simulink model "EScooter_Context_Physical"  (R2025b)
settings: Solver=VariableStepAuto  StartTime=0.0  StopTime=10.0  RelTol=1e-3
settings Model: Creator=louis  LastModifiedBy=louis

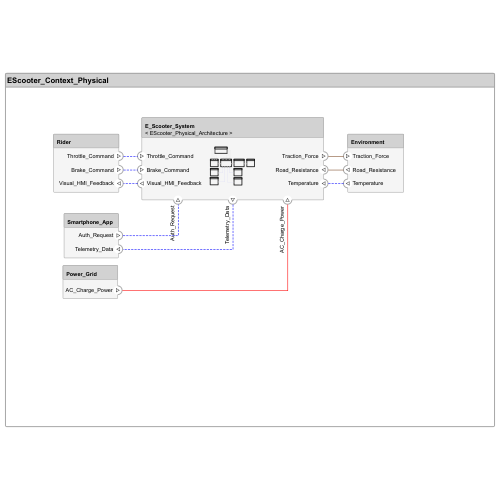
[thumbnail: Simulink's stored preview of the top-level diagram]
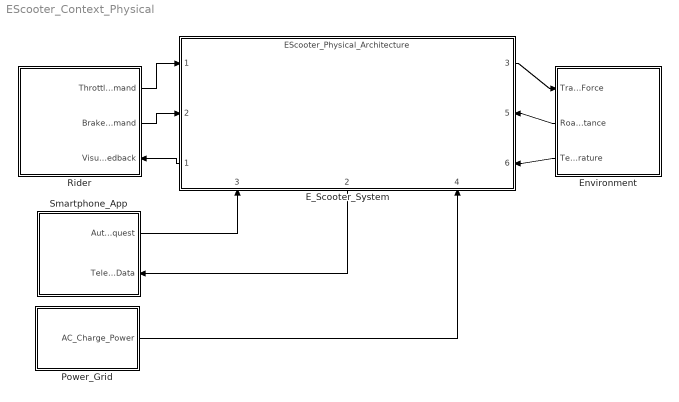
== system EScooter_Context_Physical ==
  E_Scooter_System : ModelReference  ModelNameDialog=EScooter_Physical_Architecture  SimulationMode=Normal  ModelReferenceVersion=1.35
      settings: PortSchema="{\"entries\":[{\"content\":{\"headerSize\":38,\"margin\":15,\"minimumSpacing\":25,\"sides\":[{\"content\":{\"connectorIds\":[\"In1\",\"In2\",\"Out1\"]},\"type\":\"ConnectorPlacement.EquallySpacedRectSide\",\"uuid\":\"e3bd6986-1133-4d24-a772-f86194006591\"},{\"content\":{\"connectorIds\":[\"Out3\",\"In5\",\"In6\"],\"side\":\"RIGHT\"},\"type\":\"ConnectorPlacement.EquallySpacedRectSide\",\"uuid\":\"35d8fe16-ac3e-4ad7-9024-4759d4f7a595\"},{\"content\":{\"side\":\"TOP\"},\"type\":\"ConnectorPlacement.EquallySpacedRectSide\",\"uuid\":\"5c4c1cf0-f549-46fb-a8e2-98c3709b9973\"},{\"content\":{\"connectorIds\":[\"In3\",\"Out2\",\"In4\"],\"side\":\"BOTTOM\"},\"type\":\"ConnectorPlacement.EquallySpacedRectSide\",\"uuid\":\"d5812157-23f3-4c6d-a0b8-9b10c8e876d4\"}]},\"type\":\"ConnectorPlacement.EquallySpacedConnector\",\"uuid\":\"87a80faf-9870-4a1b-94c7-6fcc75790299\"}],\"packageUris\":[\"http://schema.mathworks.com/mf0/Connector/R2020b\"],\"version\":\"1.0\"}"
  Environment : Subsystem
      settings: PortSchema="{\"entries\":[{\"content\":{\"headerSize\":26,\"margin\":15,\"minimumSpacing\":25,\"sides\":[{\"content\":{\"connectorIds\":[\"In1\",\"Out1\",\"Out2\"]},\"type\":\"ConnectorPlacement.EquallySpacedRectSide\",\"uuid\":\"144652b9-dd85-470f-8014-e792da2fa2ac\"},{\"content\":{\"side\":\"RIGHT\"},\"type\":\"ConnectorPlacement.EquallySpacedRectSide\",\"uuid\":\"d391e3f2-978f-4ccc-ab2b-52567d421a28\"},{\"content\":{\"side\":\"TOP\"},\"type\":\"ConnectorPlacement.EquallySpacedRectSide\",\"uuid\":\"a45f99b3-1281-4051-bb9b-2205db18ec2a\"},{\"content\":{\"side\":\"BOTTOM\"},\"type\":\"ConnectorPlacement.EquallySpacedRectSide\",\"uuid\":\"ad3f1504-e103-4633-a1e9-d1d529d4f8d7\"}]},\"type\":\"ConnectorPlacement.EquallySpacedConnector\",\"uuid\":\"69c8647b-5d40-4da9-a90b-a75e053ae147\"}],\"packageUris\":[\"http://schema.mathworks.com/mf0/Connector/R2020b\"],\"version\":\"1.0\"}"
  Power_Grid : Subsystem
      settings: PortSchema="{\"entries\":[{\"content\":{\"headerSize\":26,\"margin\":15,\"minimumSpacing\":25,\"sides\":[{\"content\":{},\"type\":\"ConnectorPlacement.EquallySpacedRectSide\",\"uuid\":\"144652b9-dd85-470f-8014-e792da2fa2ac\"},{\"content\":{\"connectorIds\":[\"Out1\"],\"side\":\"RIGHT\"},\"type\":\"ConnectorPlacement.EquallySpacedRectSide\",\"uuid\":\"d391e3f2-978f-4ccc-ab2b-52567d421a28\"},{\"content\":{\"side\":\"TOP\"},\"type\":\"ConnectorPlacement.EquallySpacedRectSide\",\"uuid\":\"a45f99b3-1281-4051-bb9b-2205db18ec2a\"}]},\"type\":\"ConnectorPlacement.EquallySpacedConnector\",\"uuid\":\"69c8647b-5d40-4da9-a90b-a75e053ae147\"}],\"packageUris\":[\"http://schema.mathworks.com/mf0/Connector/R2020b\"],\"version\":\"1.0\"}"
  Rider : Subsystem
      settings: PortSchema="{\"entries\":[{\"content\":{\"headerSize\":26,\"margin\":15,\"minimumSpacing\":25,\"sides\":[{\"content\":{},\"type\":\"ConnectorPlacement.EquallySpacedRectSide\",\"uuid\":\"144652b9-dd85-470f-8014-e792da2fa2ac\"},{\"content\":{\"connectorIds\":[\"Out2\",\"Out1\",\"In1\"],\"side\":\"RIGHT\"},\"type\":\"ConnectorPlacement.EquallySpacedRectSide\",\"uuid\":\"d391e3f2-978f-4ccc-ab2b-52567d421a28\"},{\"content\":{\"side\":\"TOP\"},\"type\":\"ConnectorPlacement.EquallySpacedRectSide\",\"uuid\":\"a45f99b3-1281-4051-bb9b-2205db18ec2a\"},{\"content\":{\"side\":\"BOTTOM\"},\"type\":\"ConnectorPlacement.EquallySpacedRectSide\",\"uuid\":\"8b6a9f1e-7bda-49c4-a6db-2fcaec62a930\"}]},\"type\":\"ConnectorPlacement.EquallySpacedConnector\",\"uuid\":\"69c8647b-5d40-4da9-a90b-a75e053ae147\"}],\"packageUris\":[\"http://schema.mathworks.com/mf0/Connector/R2020b\"],\"version\":\"1.0\"}"
  Smartphone_App : Subsystem
      settings: PortSchema="{\"entries\":[{\"content\":{\"headerSize\":26,\"margin\":15,\"minimumSpacing\":25,\"sides\":[{\"content\":{},\"type\":\"ConnectorPlacement.EquallySpacedRectSide\",\"uuid\":\"144652b9-dd85-470f-8014-e792da2fa2ac\"},{\"content\":{\"connectorIds\":[\"Out1\",\"In1\"],\"side\":\"RIGHT\"},\"type\":\"ConnectorPlacement.EquallySpacedRectSide\",\"uuid\":\"d391e3f2-978f-4ccc-ab2b-52567d421a28\"},{\"content\":{\"side\":\"TOP\"},\"type\":\"ConnectorPlacement.EquallySpacedRectSide\",\"uuid\":\"a45f99b3-1281-4051-bb9b-2205db18ec2a\"}]},\"type\":\"ConnectorPlacement.EquallySpacedConnector\",\"uuid\":\"69c8647b-5d40-4da9-a90b-a75e053ae147\"}],\"packageUris\":[\"http://schema.mathworks.com/mf0/Connector/R2020b\"],\"version\":\"1.0\"}"
  wires:
  Rider/2(Throttle_Command) -> E_Scooter_System/1
  Rider/1(Brake_Command) -> E_Scooter_System/2
  E_Scooter_System/1 -> Rider/1(Visual_HMI_Feedback)
  Smartphone_App/1(Auth_Request) -> E_Scooter_System/3
  E_Scooter_System/2 -> Smartphone_App/1(Telemetry_Data)
  Power_Grid/1(AC_Charge_Power) -> E_Scooter_System/4
  E_Scooter_System/3 -> Environment/1(Traction_Force)
  Environment/1(Road_Resistance) -> E_Scooter_System/5
  Environment/2(Temperature) -> E_Scooter_System/6

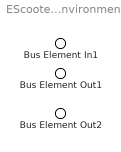
== system EScooter_Context_Physical/Environment ==
  Bus Element In1 : Inport  PortName=Traction_Force
  Bus Element Out1 : Outport  PortName=Road_Resistance
  Bus Element Out2 : Outport  Port=2  PortName=Temperature

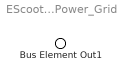
== system EScooter_Context_Physical/Power_Grid ==
  Bus Element Out1 : Outport  PortName=AC_Charge_Power

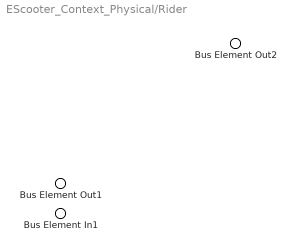
== system EScooter_Context_Physical/Rider ==
  Bus Element In1 : Inport  PortName=Visual_HMI_Feedback
  Bus Element Out2 : Outport  PortName=Brake_Command
  Bus Element Out1 : Outport  Port=2  PortName=Throttle_Command

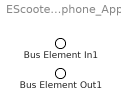
== system EScooter_Context_Physical/Smartphone_App ==
  Bus Element In1 : Inport  PortName=Telemetry_Data
  Bus Element Out1 : Outport  PortName=Auth_Request
